simulink model "tdm1"  (R2020a)
settings: Solver=VariableStepAuto  StartTime=0.0  StopTime=30  RelTol=1e-3
libraries: dsparch4 x2
settings Model: Creator=mluser  LastModifiedBy=Nitisha Singh
settings DebuggingCC: SFMachineParentedDataDiag=error

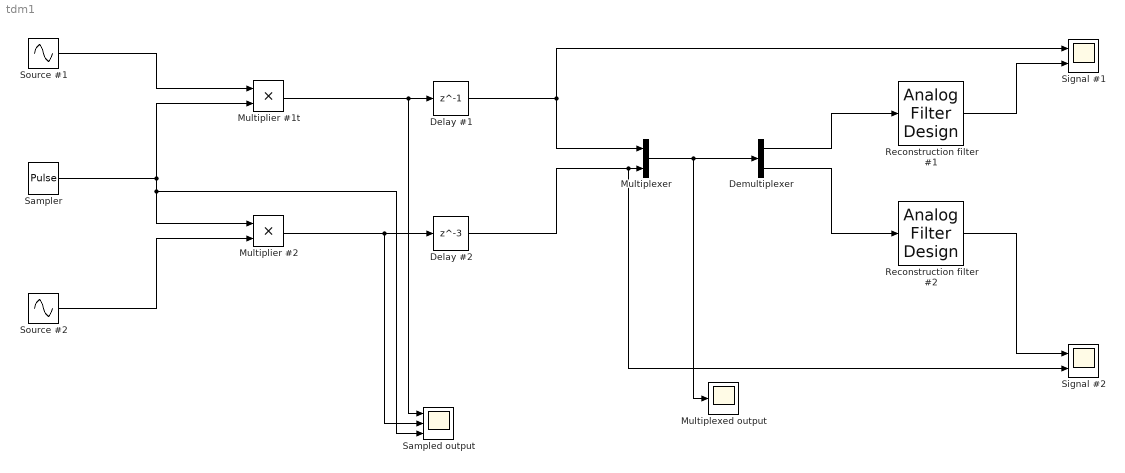
== system tdm1 ==
  Delay #1 : Delay  DelayLength=1  InitialCondition=0
  Delay #2 : Delay  DelayLength=3  InitialCondition=0
  Demultiplexer : Demux  Outputs=2
  Multiplexed output : Scope
  Multiplexer : Mux  Inputs=2
  Multiplier #1t : Product
  Multiplier #2 : Product
  Reconstruction filter #1 : dsparch4/Analog Filter Design  method=Butterworth  filttype=Lowpass  N=3  Wlo=1  Whi=80  Rp=2  Rs=40
  Reconstruction filter #2 : dsparch4/Analog Filter Design  method=Butterworth  filttype=Lowpass  N=3  Wlo=0.5  Whi=80  Rp=2  Rs=40
  Sampled output : Scope  NumInputPorts=3
  Sampler : DiscretePulseGenerator  PulseType=Time based  Period=0.5  PulseWidth=10
  Signal #1 : Scope  NumInputPorts=2
  Signal #2 : Scope  NumInputPorts=2
  Source #1 : Sin  SampleTime=0.1
  Source #2 : Sin  Frequency=0.5  SampleTime=0.1
  wires:
  Source #1/1 -> Multiplier #1t/1
  Sampler/1 -> Multiplier #2/1, Sampled output/3, Multiplier #1t/2
  Source #2/1 -> Multiplier #2/2
  Multiplier #1t/1 -> Sampled output/1, Delay #1/1
  Multiplier #2/1 -> Delay #2/1, Sampled output/2
  Delay #1/1 -> Signal #1/1, Multiplexer/1
  Delay #2/1 -> Signal #2/2, Multiplexer/2
  Multiplexer/1 -> Multiplexed output/1, Demultiplexer/1
  Demultiplexer/1 -> Reconstruction filter #1/1
  Demultiplexer/2 -> Reconstruction filter #2/1
  Reconstruction filter #1/1 -> Signal #1/2
  Reconstruction filter #2/1 -> Signal #2/1
